simulink model "rules"  (R2016a)
settings: Solver=VariableStepAuto  StartTime=0.0  StopTime=50  RelTol=1e-3
undefined symbols (not defined in the file or in its folder): DiscIntNeverNeededParam
libraries: simulink x5, fuzblock x5
settings Model: Creator=SPDKH  LastModifiedBy=SPDKH

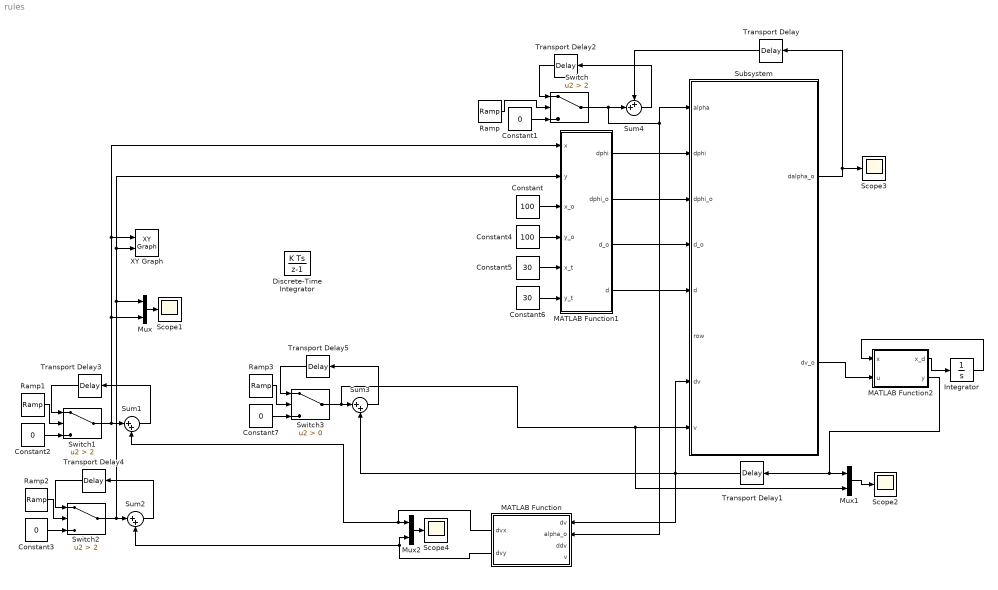
== system rules ==
  Constant : Constant  Value=100
  Constant{1..3,7} (4 alike) : Constant  Value=0
  Constant4 : Constant  Value=100
  Constant5 : Constant  Value=30
  Constant6 : Constant  Value=30
  Discrete-Time Integrator : DiscreteIntegrator  InitialConditionSetting=State (most efficient)  ICPrevOutput=DiscIntNeverNeededParam  ICPrevScaledInput=DiscIntNeverNeededParam
  Integrator : Integrator  InitialCondition=[0;0;0]
  MATLAB Function : MATLAB Function  TreatAsAtomicUnit=on
  MATLAB Function1 : MATLAB Function  TreatAsAtomicUnit=on
  MATLAB Function2 : MATLAB Function  TreatAsAtomicUnit=on
  Mux : Mux  Inputs=2
  Mux1 : Mux  Inputs=2
  Mux2 : Mux  Inputs=2
  Ramp{,1..3} (4 alike) : simulink/Sources/Ramp  slope=1  start=0  X0=0
  Scope{1..4} (4 alike) : Scope
  Subsystem : Subsystem
  Sum1 : Sum  Inputs=|++
  Sum2 : Sum  Inputs=|++
  Sum3 : Sum  Inputs=|++
  Sum4 : Sum  Inputs=++|
  Switch : Switch  Criteria=u2 > Threshold  Threshold=2
  Switch1 : Switch  Criteria=u2 > Threshold  Threshold=2
  Switch2 : Switch  Criteria=u2 > Threshold  Threshold=2
  Switch3 : Switch  Criteria=u2 > Threshold
  Transport Delay : TransportDelay  TransDelayFeedthrough=on
  Transport Delay{1,3..5} (4 alike) : TransportDelay
  Transport Delay2 : TransportDelay  TransDelayFeedthrough=on
  XY Graph : simulink/Sinks/XY Graph  xmin=-10  xmax=100  ymin=-10  ymax=100  st=-1
  wires:
  Subsystem/1("dalpha_o ") -> Scope3/1, Transport Delay/1
  Transport Delay1/1 -> Sum3/2, Subsystem/7(dv), MATLAB Function/1(dv)
  MATLAB Function1/4(d) -> Subsystem/5(d)
  MATLAB Function1/3(d_o) -> Subsystem/4(d_o)
  MATLAB Function1/2(dphi_o) -> Subsystem/3("dphi_o ")
  MATLAB Function1/1(dphi) -> Subsystem/2("dphi ")
  Constant1/1 -> Switch/3
  Ramp/1 -> Switch/2
  Constant2/1 -> Switch1/3
  Transport Delay3/1 -> Switch1/1
  Ramp1/1 -> Switch1/2
  Switch1/1 -> Mux/2, XY Graph/1, MATLAB Function1/1(x), Sum1/1
  Sum1/1 -> Transport Delay3/1
  Constant3/1 -> Switch2/3
  Transport Delay4/1 -> Switch2/1
  Ramp2/1 -> Switch2/2
  Sum2/1 -> Transport Delay4/1
  Constant/1 -> MATLAB Function1/3(x_o)
  Constant4/1 -> MATLAB Function1/4(y_o)
  Constant5/1 -> MATLAB Function1/5(x_t)
  Constant6/1 -> MATLAB Function1/6(y_t)
  Mux/1 -> Scope1/1
  Constant7/1 -> Switch3/3
  Transport Delay5/1 -> Switch3/1
  Ramp3/1 -> Switch3/2
  Sum3/1 -> Transport Delay5/1
  Switch3/1 -> Sum3/1, Subsystem/8(v), Mux1/2
  Mux1/1 -> Scope2/1
  Switch/1 -> MATLAB Function/2(alpha_o), Subsystem/1(alpha), Sum4/2
  Transport Delay/1 -> Sum4/1
  Transport Delay2/1 -> Switch/1
  MATLAB Function/2(dvy) -> Mux2/2, Sum2/2
  MATLAB Function/1(dvx) -> Sum1/2, Mux2/1
  Mux2/1 -> Scope4/1
  Sum4/1 -> Transport Delay2/1
  Switch2/1 -> Mux/1, XY Graph/2, MATLAB Function1/2(y), Sum2/1
  MATLAB Function2/1(x_d) -> Integrator/1
  Integrator/1 -> MATLAB Function2/1(x)
  Subsystem/2(dv_o) -> MATLAB Function2/2(u)
  MATLAB Function2/2(y) -> Transport Delay1/1, Mux1/1

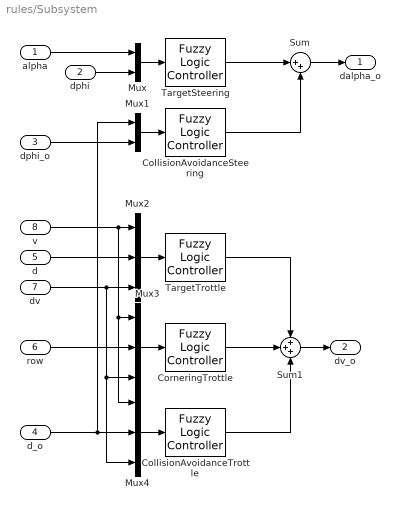
== system rules/Subsystem ==
  alpha : Inport
  "dphi " : Inport  Port=2
  "dphi_o " : Inport  Port=3
  d_o : Inport  Port=4
  d : Inport  Port=5
  row : Inport  Port=6
  dv : Inport  Port=7
  v : Inport  Port=8
  "CollisionAvoidanceSteering " : fuzblock/Fuzzy Logic  Controller  fis=['CollisionAvoidanceSteering.fis']
  "CollisionAvoidanceTrottle " : fuzblock/Fuzzy Logic  Controller  fis=['CollisionAvoidanceThrottle.fis']
  "CorneringTrottle " : fuzblock/Fuzzy Logic  Controller  fis=['CorneringTrottle.fis']
  Mux : Mux  Inputs=2
  Mux1 : Mux  Inputs=2
  Mux2 : Mux  Inputs=3
  Mux3 : Mux  Inputs=3
  Mux4 : Mux  Inputs=3
  Sum : Sum  Inputs=|++
  Sum1 : Sum  Inputs=+++
  TargetSteering : fuzblock/Fuzzy Logic  Controller  fis=['TargetSteering2.fis']
  TargetTrottle : fuzblock/Fuzzy Logic  Controller  fis=['TargetTrottle.fis']
  "dalpha_o " : Outport
  dv_o : Outport  Port=2
  wires:
  TargetTrottle/1 -> Sum1/1
  "CorneringTrottle "/1 -> Sum1/2
  "CollisionAvoidanceTrottle "/1 -> Sum1/3
  TargetSteering/1 -> Sum/1
  "CollisionAvoidanceSteering "/1 -> Sum/2
  Mux/1 -> TargetSteering/1
  Mux1/1 -> "CollisionAvoidanceSteering "/1
  Mux2/1 -> TargetTrottle/1
  Mux3/1 -> "CorneringTrottle "/1
  Mux4/1 -> "CollisionAvoidanceTrottle "/1
  v/1 -> Mux4/1, Mux3/1, Mux2/1
  d/1 -> Mux2/2
  dv/1 -> Mux4/3, Mux3/3, Mux2/3
  row/1 -> Mux3/2
  d_o/1 -> Mux1/1, Mux4/2
  alpha/1 -> Mux/1
  "dphi "/1 -> Mux/2
  "dphi_o "/1 -> Mux1/2
  Sum/1 -> "dalpha_o "/1
  Sum1/1 -> dv_o/1

== matlab function rules/MATLAB Function1 ==
  data: dphi output; dphi_o output; d_o output; x input; d output; y input; x_o input; y_o input; x_t input; y_t input
function [dphi,dphi_o,d_o,d] = fcn(x,y,x_o,y_o,x_t,y_t)
%#codegen
if (((y_t-y)<0 && (x_t-x)>0)||((y_t-y)<0 && (x_t-x)<0))
    dphi = atan ((y_t-y)/(x_t-x))+pi;
else 
    dphi = atan ((y_t-y)/(x_t-x));
end
dphi_o = atan ((y_o-y)/(x_o-x));

d_o = norm([(x_o-x),(y_o-y)]);
d = norm([(x_t-x),(y_t-y)]);

== matlab function rules/MATLAB Function ==
  data: dv input; dvx output; alpha_o input; dvy output; ddv input; v input
function [dvx,dvy] = fcn(dv,alpha_o,ddv,v)
%#codegen

dvx = dv*cos(alpha_o);
dvy = dv*sin(alpha_o);

% ddvx = ddv*cos(alpha_o);
% ddvy = ddv*sin(alpha_o);
% row = v^3 / abs((dvx*dvy)-(dvy*ddvx));

== matlab function rules/MATLAB Function2 ==
  data: x input; u input; x_d output; y output
function [x_d,y]= fcn(x,u)

A = [-6.0476 -5.2856 -0.2380;1.0000 0 0; 0 1.0000 0];
B =[1 0 0]';
C =[0 0 2.4767];

x_d = A*x +B*u;
y = C*x;
